simulink model "UsartControl"  (R2016a)
settings: Solver=FixedStepAuto  StartTime=0.0  StopTime=inf  FixedStep=0.001  RelTol=1e-3
undefined symbols (not defined in the file): serial
libraries: instrumentlib x3, simulink x1
settings Model: Creator=LMPC  LastModifiedBy=LMPC

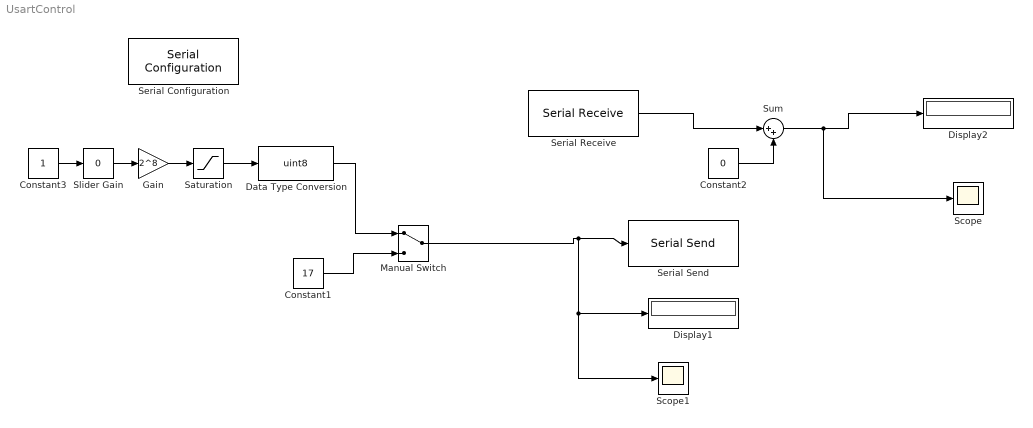
== system UsartControl ==
  Constant1 : Constant  Value=17  OutDataTypeStr=uint8  SampleTime=-1
  Constant2 : Constant  Value=0  OutDataTypeStr=uint8  SampleTime=-1
  Constant3 : Constant  OutDataTypeStr=single  SampleTime=-1
  Data Type Conversion : DataTypeConversion  OutDataTypeStr=uint8
  Display1 : Display
      settings: Format=hex (Stored Integer)
  Display2 : Display
      settings: Format=hex (Stored Integer)
  Gain : Gain  Gain=2^8
  Manual Switch : ManualSwitch
  Saturation : Saturate  UpperLimit=2^8-1  LowerLimit=0
  Scope : Scope
  Scope1 : Scope
  Serial Configuration : instrumentlib/Serial Configuration  Priority=-200000  ComPortMenu=COM1  ComPort=COM1  ObjConstructor=serial('COM1');  BaudRate=57600  DataBits=8  Parity=none  StopBits=1  FlowControl=none  Timeout=10  ByteOrder=LittleEndian
  Serial Receive : instrumentlib/Serial Receive  ComPortMenu=COM1  ComPort=COM1  ObjConstructor=serial('COM1');  Terminator=<none>  DataSize=1  DataType=uint8  EnableBlockingMode=on  ActionDataUnavailable=Output custom value  CustomValue=-25  SampleTime=0.001
  Serial Send : instrumentlib/Serial Send  ComPortMenu=COM1  ComPort=COM1  ObjConstructor=serial('COM1');  Terminator=<none>  EnableBlockingMode=off
  Slider Gain : simulink/Math Operations/Slider Gain  low=0  gain=0  high=1
  Sum : Sum  Inputs=|++
  wires:
  Manual Switch/1 -> Scope1/1, Display1/1, Serial Send/1
  Constant1/1 -> Manual Switch/2
  Sum/1 -> Scope/1, Display2/1
  Constant2/1 -> Sum/2
  Serial Receive/1 -> Sum/1
  Gain/1 -> Saturation/1
  Slider Gain/1 -> Gain/1
  Constant3/1 -> Slider Gain/1
  Data Type Conversion/1 -> Manual Switch/1
  Saturation/1 -> Data Type Conversion/1
